simulink model "ADIA"  (R2018b)
settings: Solver=FixedStepDiscrete  StartTime=0.0  StopTime=10.0  FixedStep=0.02  RelTol=1e-3
undefined symbols (not defined in the file or in its folder): ACC_State_Active, ACC_State_BrakeOnly, ACC_State_Suspended, ACC_State_WaitingRise, ADAS_AEBBrakingProg, ADAS_DeclControlReq, ADAS_DriveOff, ADAS_ESCHoldReq_NotHold, ADASDecType_ACC, ADASDecType_AEB, ADIA_ACC_Acceleration_OOR_DecCount_C, ADIA_ACC_Acceleration_OOR_Duration_C, ADIA_ACC_Acceleration_OOR_IncCount_C, ADIA_ACC_Acceleration_OOR_LLim_C, ADIA_ACC_Acceleration_OOR_ULim_C, ADIA_ACC_AccelTrqReq_MixedDia_ULim_C, ADIA_ACC_AccelTrqReq_ULim_C, ADIA_ACC_Deceleration_Mixed_ULim_C, ADIA_ACC_Deceleration_OOR_DecCount_C, ADIA_ACC_Deceleration_OOR_Duration_C, ADIA_ACC_Deceleration_OOR_IncCount_C, ADIA_ACC_Deceleration_OOR_LLim_C, ADIA_ACC_Deceleration_OOR_ULim_C, ADIA_ACC_DriveOff_Distance_C, ADIA_ACC_DriveOff_TimeLim_C, ADIA_ACC_ReqMixed_DecCount_C, ADIA_ACC_ReqMixed_Duration_C, ADIA_ACC_ReqMixed_IncCount_C, ADIA_AccPedalRaw_MaxLim_C, ADIA_AccPedalRaw_MinLim_C, ADIA_ADAS_HoldDecReq_Set_C, ADIA_ADAS_HoldRConfirm_TimeLim_C, ADIA_ADAS_HoldVehSpd_Lim_C, ADIA_AEB_VehSpdDec_LLim_C, ADIA_AEB_VehSpdDec_ULim_C, ADIA_ASWFault_OvrdEn_C, ADIA_ASWFault_OvrdValue_C, ADIA_BatteryOutOfRange_DecCount_C, ADIA_BatteryOutOfRange_Duration_C, ADIA_BatteryOutOfRange_IncCount_C, ADIA_BattVolt_MaxLim_C, ADIA_BattVolt_MinLim_C, ADIA_BCM3_33C_InvBrkLight_DecCount_C, ADIA_BCM3_33C_InvBrkLight_Duration_C, ADIA_BCM3_33C_InvBrkLight_IncCount_C, ADIA_BCM_BattVolt_OvrdEn_C, ADIA_BCM_BattVolt_OvrdVal_C, ADIA_BCM_BrakeLampStaus_OvrdEn_C, ADIA_BCM_BrakeLampStaus_OvrdVal_C, ADIA_BCM_CHMSLStaus_OvrdEn_C, ADIA_BCM_CHMSLStaus_OvrdVal_C, ADIA_BCM_LeftTurnSwSt_OvrdEn_C, ADIA_BCM_LeftTurnSwSt_OvrdVal_C, ADIA_BCM_RightTurnSwSt_OvrdEn_C, ADIA_BCM_RightTurnSwSt_OvrdVal_C, ADIA_BCM_TurnSwFailure_DecCount_C, ADIA_BCM_TurnSwFailure_Duration_C, ADIA_BCM_TurnSwFailure_IncCount_C, ADIA_BSWFault_Ignore_C, ADIA_BSWFault_OvrdEn_C ... (+281)
libraries: simulink x208
(part 2 of 10)

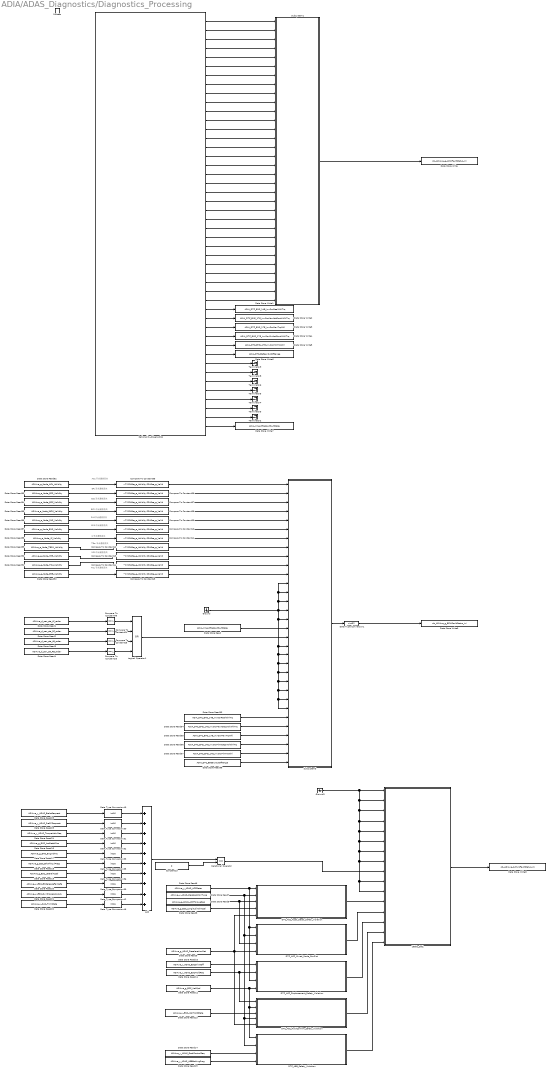
== system ADIA/ADAS_Diagnostics/Diagnostics_Processing ==
  note: ESC节点通信丢失
  note: TCU节点通信丢失
  note: EPS节点通信丢失
  note: ACU节点通信丢失
  note: MP5节点通信丢失
  note: EMS节点通信丢失
  note: TBox节点通信丢失
  note: IC节点通信丢失
  note: BCM节点通信丢失
  note: SAS节点通信丢失
  Process : TriggerPort  TriggerType=function-call  VariantControl=(inherit)
  16Bits_Set1 : Subsystem
  Add : Sum  Inputs=++++++++++
  Compare To Constant{24..26,48} (4 alike) : simulink/Logic and Bit Operations/Compare To Constant  relop===  const=1  OutDataTypeStr=boolean
  Compare To Constant{35..45} (11 alike) : simulink/Logic and Bit Operations/Compare To Constant  relop=~=  const=SPARte_e_Validity.SPARce_e_Valid  OutDataTypeStr=boolean
  Constant13 : Constant  Value=0  OutDataTypeStr=int16
  DTC_ACC_Accel_Decel_Safety_Violation : Subsystem
  DTC_ACC_Displacement_Safety_Violation : Subsystem
  DTC_ACC_HoldConfirm_Safety_Violation : Subsystem
  DTC_ACC_Mixed_Mode_Conflict : Subsystem
  DTC_AEB_Safety_Violation : Subsystem
  Data Store Read : DataStoreRead  DataStoreName=ADIA_Inner_FRadar_FaultState
  Data Store Read1 : DataStoreRead  DataStoreName=ADIAve_d_sen_sta_LF_radar
  Data Store Read10 : DataStoreRead  DataStoreName=ADIAve_y_ADAS_ESCDriveOff
  Data Store Read11 : DataStoreRead  DataStoreName=ADIAve_y_ADAS_ESCHoldReq
  Data Store Read12 : DataStoreRead  DataStoreName=ADIAve_g_ESC_VehSpd
  Data Store Read13 : DataStoreRead  DataStoreName=ADIAve_y_ESC_VehHoldState
  Data Store Read14 : DataStoreRead  DataStoreName=ADIAve_y_ADAS_DeclControlReq
  Data Store Read15 : DataStoreRead  DataStoreName=ADIAve_y_ADAS_AEBBrakingProg
  Data Store Read16 : DataStoreRead  DataStoreName=ADIAve_g_EMS_AccPedalPos
  Data Store Read17 : DataStoreRead  DataStoreName=ADIAve_g_EMS_EngIndTrq
  Data Store Read18 : DataStoreRead  DataStoreName=ADIAve_g_ESC_BrkWhlCylPress
  Data Store Read19 : DataStoreRead  DataStoreName=ADIAve_g_ESC_LateralAccel
  Data Store Read2 : DataStoreRead  DataStoreName=ADIAve_d_sen_sta_RF_radar
  Data Store Read20 : DataStoreRead  DataStoreName=ADIAve_y_ESC_BrkReleaseFailsafe
  Data Store Read21 : DataStoreRead  DataStoreName=ADIAve_y_ESC_DynSlopeAccuracy
  Data Store Read22 : DataStoreRead  DataStoreName=ADIAve_y_SAS_TrimState
  Data Store Read23 : DataStoreRead  DataStoreName=ADIAve_y_ADAS_PrefillRequest
  Data Store Read24 : DataStoreRead  DataStoreName=ADIAve_y_ADAS_TorqueActivReq
  Data Store Read25 : DataStoreRead  DataStoreName=ADIAve_y_ADAS_BrakeRequest
  Data Store Read3 : DataStoreRead  DataStoreName=ADIAve_d_sen_sta_LB_radar
  Data Store Read4 : DataStoreRead  DataStoreName=ADIAve_d_sen_sta_RB_radar
  Data Store Read5 : DataStoreRead  DataStoreName=ADIAve_g_ADAS_ACCTorqueReq
  Data Store Read6 : DataStoreRead  DataStoreName=ADIAve_y_ADAS_ACCState
  Data Store Read7 : DataStoreRead  DataStoreName=ADIAve_y_ADAS_DecelerationType
  Data Store Read8 : DataStoreRead  DataStoreName=ADIAve_g_ESC_LongitudinalAccel
  Data Store Read82 : DataStoreRead  DataStoreName=ADIAve_e_Node_ACU_Validity
  Data Store Read83 : DataStoreRead  DataStoreName=ADIAve_e_Node_EPS_Validity
  Data Store Read84 : DataStoreRead  DataStoreName=ADIAve_e_Node_ESC_Validity
  Data Store Read85 : DataStoreRead  DataStoreName=ADIAve_e_Node_IBCM_Validity
  Data Store Read86 : DataStoreRead  DataStoreName=ADIAve_e_Node_SAS_Validity
  Data Store Read87 : DataStoreRead  DataStoreName=ADIAve_e_Node_EMS_Validity
  Data Store Read88 : DataStoreRead  DataStoreName=ADIAve_e_Node_IC_Validity
  Data Store Read89 : DataStoreRead  DataStoreName=ADIAve_e_Node_TBOX_Validity
  Data Store Read9 : DataStoreRead  DataStoreName=ADIAve_g_ADAS_DecelerationSet
  Data Store Read90 : DataStoreRead  DataStoreName=ADIAve_e_Node_MP5_Validity
  Data Store Read91 : DataStoreRead  DataStoreName=ADIAve_e_Node_TCU_Validity
  Data Store Read92 : DataStoreRead  DataStoreName=ADIAve_e_Node_EPB_Validity
  Data Store Read93 : DataStoreRead  DataStoreName=ADIA_DTC_EMS_14B_InvOorRealWhlTrq
  Data Store Read94 : DataStoreRead  DataStoreName=ADIA_DTC_EMS_17E_InvOorMaxNotContrlWhlTrq
  Data Store Read95 : DataStoreRead  DataStoreName=ADIA_DTC_EMS_17E_InvOorMaxTrqWhl
  Data Store Read96 : DataStoreRead  DataStoreName=ADIA_DTC_EMS_17E_InvOorMinNotContrlWhlTrq
  Data Store Read97 : DataStoreRead  DataStoreName=ADIA_DTC_EMS_17E_InvOorMinTrqWhl
  Data Store Read98 : DataStoreRead  DataStoreName=ADIA_DTC_BatteryOutOfRange
  Data Store Write : DataStoreWrite  DataStoreName=ob_ADIAve_g_ASWFaultStatus_ini
  Data Store Write1 : DataStoreWrite  DataStoreName=ADIA_DTC_EMS_14B_InvOorRealWhlTrq
  Data Store Write2 : DataStoreWrite  DataStoreName=ADIA_DTC_EMS_17E_InvOorMaxNotContrlWhlTrq
  Data Store Write3 : DataStoreWrite  DataStoreName=ADIA_DTC_EMS_17E_InvOorMaxTrqWhl
  Data Store Write4 : DataStoreWrite  DataStoreName=ADIA_DTC_EMS_17E_InvOorMinNotContrlWhlTrq
  Data Store Write5 : DataStoreWrite  DataStoreName=ADIA_DTC_EMS_17E_InvOorMinTrqWhl
  Data Store Write6 : DataStoreWrite  DataStoreName=ADIA_DTC_BatteryOutOfRange
  Data Store Write7 : DataStoreWrite  DataStoreName=ADIA_Inner_FRadar_FaultState
  Data Store Write8 : DataStoreWrite  DataStoreName=ob_ADIAve_d_FuncFaultStatus_ini
  Data Store Write9 : DataStoreWrite  DataStoreName=ob_ADIAve_g_BSWFaultStatus_ini
  Data Type Conversion1 : DataTypeConversion  OutDataTypeStr=uint32
  Data Type Conversion{30..33,35..36,39,42,46,49} (10 alike) : DataTypeConversion  OutDataTypeStr=int16
  Ground : Ground
  Ground3 : Ground
  Logical Operator1 : Logic  Operator=OR  Inputs=4  AllPortsSameDT=off  OutDataTypeStr=boolean
  Rationality_Diagnostics : Subsystem
  Relational Operator : RelationalOperator  Operator===  OutDataTypeStr=boolean  RndMeth=Simplest
  Subsystem1 : Subsystem
  Subsystem3 : Subsystem
  Terminator{2..6,8..9} (7 alike) : Terminator
  wires:
  Rationality_Diagnostics/46(ADIA_Inner_FRadar_FaultState) -> Data Store Write7/1
  Data Store Read95/1 -> Subsystem3/29(Bit28)
  Data Store Read94/1 -> Subsystem3/28(Bit27)
  Rationality_Diagnostics/3(ADIA_DTC_SAS_SASFailureSts) -> Subsystem1/3(Bit2)
  Ground/1 -> Subsystem3/26(Bit25), Subsystem3/25(Bit24), Subsystem3/24(Bit23), Subsystem3/23(Bit22), Subsystem3/22(Bit21), Subsystem3/21(Bit20), Subsystem3/20(Bit19), Subsystem3/19(Bit18), Subsystem3/16(Bit15), Subsystem3/12(Bit11), Subsystem3/13(Bit12), Subsystem3/14(Bit13), Subsystem3/15(Bit14)
  Rationality_Diagnostics/34(ADIA_DTC_EMS_17E_InvOorMaxNotContrlWhlTrq) -> Data Store Write2/1
  Data Store Read97/1 -> Subsystem3/31(Bit30)
  Data Store Read92/1 -> Compare To Constant45/1
  Data Store Read98/1 -> Subsystem3/32(Bit31)
  Compare To Constant43/1 -> Subsystem3/9(Bit8)  "Event_OutRangePowStrSta_SetEventStatus19"
  Data Store Read/1 -> Subsystem3/17(Bit16)
  Data Store Read6/1 -> DTC_ACC_Mixed_Mode_Conflict/1(ADIAve_y_ADAS_ACCState), DTC_ACC_Displacement_Safety_Violation/3(ADIAve_y_ADAS_ACCState), DTC_ACC_Accel_Decel_Safety_Violation/1(ADIAve_y_ADAS_ACCState)
  Rationality_Diagnostics/43(Event_OutRangeEPSLKASta_SetEventStatus18) -> Terminator4/1
  Rationality_Diagnostics/44(Event_OutRangePowStrSta_SetEventStatus7) -> Terminator3/1
  Data Store Read3/1 -> Compare To Constant25/1
  Data Store Read14/1 -> DTC_AEB_Safety_Violation/3(ADIAve_y_ADAS_DeclControlReq)
  Data Store Read96/1 -> Subsystem3/30(Bit29)
  Data Store Read16/1 -> Data Type Conversion32/1
  Rationality_Diagnostics/38(ADIA_DTC_BatteryOutOfRange) -> Data Store Write6/1
  Rationality_Diagnostics/2(ADIA_DTC_ESC_EPBErrorStatus) -> Subsystem1/2(Bit1)
  Rationality_Diagnostics/33(ADIA_DTC_EMS_14B_InvOorRealWhlTrq) -> Data Store Write1/1
  Rationality_Diagnostics/39(Event_FaultATFail) -> Terminator9/1
  Compare To Constant36/1 -> Subsystem3/2(Bit1)  "Event_OutRangePowStrSta_SetEventStatus19"
  Data Store Read25/1 -> Data Type Conversion49/1
  Compare To Constant39/1 -> Subsystem3/5(Bit4)  "Event_OutRangePowStrSta_SetEventStatus19"
  Rationality_Diagnostics/37(ADIA_DTC_EMS_17E_InvOorMinTrqWhl) -> Data Store Write5/1
  Data Store Read93/1 -> Subsystem3/27(Bit26)
  Data Store Read12/1 -> DTC_ACC_Displacement_Safety_Violation/4(ADIAve_g_ESC_VehSpd), DTC_AEB_Safety_Violation/1(ADIAve_g_ESC_VehSpd), DTC_ACC_HoldConfirm_Safety_Violation/2(ADIAve_g_ESC_VehSpd)
  Rationality_Diagnostics/11(ADIA_DTC_EPS2_17A_InvStTorq) -> Subsystem1/11(Bit10)
  Data Store Read9/1 -> DTC_ACC_HoldConfirm_Safety_Violation/5(ADIAve_g_ADAS_DecelerationSet), DTC_ACC_Accel_Decel_Safety_Violation/5(ADIAve_g_ADAS_DecelerationSet), DTC_ACC_Mixed_Mode_Conflict/4(ADIAve_g_ADAS_DecelerationSet)
  Rationality_Diagnostics/41(Event_OutRangePowStrSta_SetEventStatus19) -> Terminator6/1
  Data Store Read10/1 -> DTC_ACC_Displacement_Safety_Violation/1(ADIAve_y_ADAS_ESCDriveOff)
  Rationality_Diagnostics/35(ADIA_DTC_EMS_17E_InvOorMaxTrqWhl) -> Data Store Write3/1
  Rationality_Diagnostics/36(ADIA_DTC_EMS_17E_InvOorMinNotContrlWhlTrq) -> Data Store Write4/1
  Rationality_Diagnostics/42(Event_FaulEPSLKASta_SetEventStatus17) -> Terminator5/1
  Data Store Read5/1 -> DTC_ACC_Mixed_Mode_Conflict/3(ADIAve_g_ADAS_ACCTorqueReq), DTC_ACC_Accel_Decel_Safety_Violation/3(ADIAve_g_ADAS_ACCTorqueReq)
  Rationality_Diagnostics/40("Event_Fault_ABSorESC ") -> Terminator8/1
  Rationality_Diagnostics/45(Event_OutRangePowStrSta_SetEventStatus9) -> Terminator2/1
  Ground3/1 -> 16Bits_Set1/1(Bit0), 16Bits_Set1/2(Bit1), 16Bits_Set1/3(Bit2), 16Bits_Set1/4(Bit3), 16Bits_Set1/5(Bit4), 16Bits_Set1/7(Bit6), 16Bits_Set1/8(Bit7), 16Bits_Set1/10(Bit9), 16Bits_Set1/11(Bit10), 16Bits_Set1/6(Bit5)
  Rationality_Diagnostics/5(ADIA_DTC_BCM3_33C_InvBrkLight) -> Subsystem1/5(Bit4)
  Rationality_Diagnostics/32(ADIA_DTC_CameraSystemError) -> Subsystem1/32(Bit31)
  Compare To Constant35/1 -> Subsystem3/1(Bit0)  "Event_OutRangePowStrSta_SetEventStatus19"
  Compare To Constant26/1 -> Logical Operator1/4
  DTC_ACC_Mixed_Mode_Conflict/1(ADIA_DTC_ACC_Mixed_Mode_Conflict) -> 16Bits_Set1/13(Bit12)  "ob_DTC_ACC_Mixed_Mode_Conflict"
  Constant13/1 -> Relational Operator/2
  DTC_ACC_HoldConfirm_Safety_Violation/1(ADIA_DTC_ACC_HoldConfirm_Safety_Violation) -> 16Bits_Set1/15(Bit14)  "ob_DTC_ACC_HoldConfirm_Safety_Violation"
  Data Type Conversion46/1 -> Add/10
  Data Type Conversion33/1 -> Add/5
  Compare To Constant40/1 -> Subsystem3/6(Bit5)  "Event_OutRangePowStrSta_SetEventStatus19"
  Data Type Conversion42/1 -> Add/9
  Compare To Constant42/1 -> Subsystem3/8(Bit7)  "Event_OutRangePowStrSta_SetEventStatus19"
  Compare To Constant44/1 -> Subsystem3/10(Bit9)  "Event_OutRangePowStrSta_SetEventStatus19"
  Data Type Conversion49/1 -> Add/1
  Compare To Constant41/1 -> Subsystem3/7(Bit6)  "Event_OutRangePowStrSta_SetEventStatus19"
  DTC_ACC_Displacement_Safety_Violation/1(ADIA_DTC_ACC_Displacement_Safety_Violation) -> 16Bits_Set1/14(Bit13)  "ob_DTC_ACC_Displacement_Safety_Violation"
  Data Type Conversion39/1 -> Add/8
  Rationality_Diagnostics/17(ADIA_DTC_ESC5_122_InvOorLongiAccel) -> Subsystem1/17(Bit16)
  Rationality_Diagnostics/7(ADIA_DTC_EMS10_88_InvAccPedPosRaw) -> Subsystem1/7(Bit6)
  Rationality_Diagnostics/8(ADIA_DTC_EMS5_E0_InvOorBrkPedal) -> Subsystem1/8(Bit7)
  Rationality_Diagnostics/25(ADIA_DTC_GW_MP5_413_OorLKAMode) -> Subsystem1/25(Bit24)
  Compare To Constant38/1 -> Subsystem3/4(Bit3)  "Event_OutRangePowStrSta_SetEventStatus19"
  Rationality_Diagnostics/16(ADIA_DTC_ESC5_122_InvOorLatAccel) -> Subsystem1/16(Bit15)
  Rationality_Diagnostics/13(ADIA_DTC_ESC2_A0_InvOorVehSpeed) -> Subsystem1/13(Bit12)
  Rationality_Diagnostics/9(ADIA_DTC_EMS5_E0_OorEngineStas) -> Subsystem1/9(Bit8)
  Rationality_Diagnostics/15(ADIA_DTC_ESC3_121_InvOorVehStandstill) -> Subsystem1/15(Bit14)
  Compare To Constant45/1 -> Subsystem3/11(Bit10)  "Event_OutRangePowStrSta_SetEventStatus19"
  Rationality_Diagnostics/22(ADIA_DTC_ESC6_123_InvVehDriDirec) -> Subsystem1/22(Bit21)
  Rationality_Diagnostics/12(ADIA_DTC_EPS3_31C_InvOorLKAState) -> Subsystem1/12(Bit11)
  Rationality_Diagnostics/6(ADIA_DTC_EMS_14A_OorACCStatus) -> Subsystem1/6(Bit5)
  Data Store Read2/1 -> Compare To Constant24/1
  Rationality_Diagnostics/27(ADIA_DTC_MP5_366_OorFCWButton) -> Subsystem1/27(Bit26)
  Data Type Conversion31/1 -> Add/3
  Compare To Constant24/1 -> Logical Operator1/2
  Compare To Constant25/1 -> Logical Operator1/3
  Rationality_Diagnostics/4(ADIA_DTC_BCM_TurnSwFailure) -> Subsystem1/4(Bit3)
  Subsystem3/1(Index_32Bits) -> Data Type Conversion1/1
  Rationality_Diagnostics/26(ADIA_DTC_MP5_366_OorAEBButton) -> Subsystem1/26(Bit25)
  Rationality_Diagnostics/1(ADIA_DTC_WheelSpdFaultSignal) -> Subsystem1/1(Bit0)
  Data Store Read23/1 -> Data Type Conversion30/1
  DTC_AEB_Safety_Violation/1(DTC_AEB_Safety_Violation) -> 16Bits_Set1/16(Bit15)  "ob_DTC_AEB_Safety_Violation"
  Data Store Read8/1 -> DTC_ACC_Accel_Decel_Safety_Violation/4(ADIAve_g_ESC_LongitudinalAccel)
  Data Store Read19/1 -> Data Type Conversion36/1
  Data Store Read13/1 -> DTC_ACC_HoldConfirm_Safety_Violation/3(ADIAve_y_ESC_VehHoldState)
  Rationality_Diagnostics/29(ADIA_DTC_SAS_A5_InvRotSpeed) -> Subsystem1/29(Bit28)
  Data Store Read21/1 -> Data Type Conversion42/1
  Data Store Read22/1 -> Data Type Conversion46/1
  Rationality_Diagnostics/18(ADIA_DTC_ESC5_122_InvOorStaticSlope) -> Subsystem1/18(Bit17)
  Rationality_Diagnostics/30(ADIA_DTC_SCC_309_OorACCButton) -> Subsystem1/30(Bit29)
  Add/1 -> Relational Operator/1
  Data Type Conversion35/1 -> Add/6
  Rationality_Diagnostics/19(ADIA_DTC_ESC5_122_InvOorYawRate) -> Subsystem1/19(Bit18)
  Data Store Read20/1 -> Data Type Conversion39/1
  Data Store Read7/1 -> DTC_ACC_HoldConfirm_Safety_Violation/4(ADIAve_y_ADAS_DecelerationType), DTC_AEB_Safety_Violation/2(ADIAve_y_ADAS_DecelerationType), DTC_ACC_Mixed_Mode_Conflict/2(ADIAve_y_ADAS_DecelerationType), DTC_ACC_Accel_Decel_Safety_Violation/2(ADIAve_y_ADAS_DecelerationType)
  Data Type Conversion1/1 -> Data Store Write9/1  "ob_ADIAve_d_BSWFaultStatus_ini"
  Compare To Constant37/1 -> Subsystem3/3(Bit2)  "Event_OutRangePowStrSta_SetEventStatus19"
  Rationality_Diagnostics/28(ADIA_DTC_SAS_A5_InvOorSteAngle) -> Subsystem1/28(Bit27)
  Data Type Conversion36/1 -> Add/7
  Data Store Read15/1 -> DTC_AEB_Safety_Violation/4(ADIAve_y_ADAS_AEBBrakingProg)
  DTC_ACC_Accel_Decel_Safety_Violation/1(ADIA_DTC_ACC_Accel_Decel_Safety_Violation) -> 16Bits_Set1/12(Bit11)  "ob_DTC_ACC_Accel_Decel_Safety_Violation"
  Logical Operator1/1 -> Subsystem3/18(Bit17)
  Data Store Read11/1 -> DTC_ACC_HoldConfirm_Safety_Violation/1(ADIAve_y_ADAS_ESCHoldReq), DTC_ACC_Displacement_Safety_Violation/2(ADIAve_y_ADAS_ESCHoldReq)
  Data Store Read90/1 -> Compare To Constant43/1
  Data Store Read91/1 -> Compare To Constant44/1
  Rationality_Diagnostics/24(ADIA_DTC_GW_MP5_413_OorISAMode) -> Subsystem1/24(Bit23)
  Rationality_Diagnostics/10(ADIA_DTC_EPS2_17A_InvOorSteAngle) -> Subsystem1/10(Bit9)
  Data Store Read87/1 -> Compare To Constant40/1
  Data Store Read86/1 -> Compare To Constant39/1
  Data Store Read85/1 -> Compare To Constant38/1
  Data Store Read83/1 -> Compare To Constant36/1
  Data Store Read17/1 -> Data Type Conversion33/1
  Rationality_Diagnostics/31(ADIA_DTC_TCU1_93_InvOorGear) -> Subsystem1/31(Bit30)
  Data Store Read82/1 -> Compare To Constant35/1
  Compare To Constant48/1 -> Logical Operator1/1
  Rationality_Diagnostics/20(ADIA_DTC_ESC6_123_InvOorDynSlope) -> Subsystem1/20(Bit19)
  Data Store Read18/1 -> Data Type Conversion35/1
  Data Type Conversion30/1 -> Add/2
  Data Store Read89/1 -> Compare To Constant42/1
  Data Store Read84/1 -> Compare To Constant37/1
  Rationality_Diagnostics/14(ADIA_DTC_ESC3_121_InvOorTCSActive) -> Subsystem1/14(Bit13)
  Data Type Conversion32/1 -> Add/4
  Rationality_Diagnostics/23(ADIA_DTC_ESC6_123_InvVehHoldStas) -> Subsystem1/23(Bit22)
  Data Store Read1/1 -> Compare To Constant48/1
  16Bits_Set1/1(Index_16Bits) -> Data Store Write8/1  "ob_ADIAve_d_FuncFaultStatus_ini"
  Data Store Read88/1 -> Compare To Constant41/1
  Rationality_Diagnostics/21(ADIA_DTC_ESC6_123_InvUnfilYawRate) -> Subsystem1/21(Bit20)
  Data Store Read24/1 -> Data Type Conversion31/1
  Data Store Read4/1 -> Compare To Constant26/1
  Subsystem1/1(Index_32Bits) -> Data Store Write/1  "ob_ADIAve_d_BSWFaultStatus_ini"
  Relational Operator/1 -> 16Bits_Set1/9(Bit8)  "ob_ADIA_SpareDataCheck"
